simulink model "lab2addingzero"  (R2014a)
settings: Solver=ode45  StartTime=0.0  StopTime=3.0  MaxStep=.001  RelTol=1e-3
values from neighbouring files (symbols this model uses):
  z = .6    (= 0.6)    [lab2code.m]
settings Model: Creator=mmroman2  LastModifiedBy=Matthew
settings DataIOCC: LimitDataPoints=off

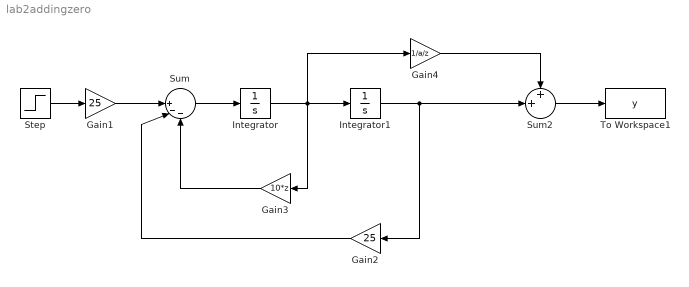
== system lab2addingzero ==
  Gain1 : Gain  Gain=25
  Gain2 : Gain  Gain=25
  Gain3 : Gain  Gain=10*z
  Gain4 : Gain  Gain=1/a/z
  Integrator : Integrator
  Integrator1 : Integrator
  Step : Step  Time=0  SampleTime=0
  Sum : Sum  Inputs=||+--
  Sum2 : Sum  Inputs=++|
  To Workspace1 : ToWorkspace  VariableName=y  SampleTime=-1
  wires:
  Step/1 -> Gain1/1
  Gain1/1 -> Sum/1
  Gain2/1 -> Sum/2
  Gain3/1 -> Sum/3
  Sum/1 -> Integrator/1
  Integrator/1 -> Gain4/1, Gain3/1, Integrator1/1
  Gain4/1 -> Sum2/1
  Integrator1/1 -> Sum2/2, Gain2/1
  Sum2/1 -> To Workspace1/1
